simulink model "Model_TranslationEngine64"  (R2022b)
settings: Solver=FixedStepDiscrete  StartTime=0.0  StopTime=5  RelTol=1e-3  EnableMultiTasking=on
InitFcn:
  | % Initialize model
  | ModelSettings=BTConfig.GetModelSettings();
  | 
  | ModelSettings.Validate();
  | 
  | ModelInit;
  | 
  | 
  | % load library data
  | GainLibrary_data;
  | % Load saved values from partition process
  | CapturedConstMask.LoadMapFromFile(bdroot)
StartFcn:
  | % make sure all the simulated RTC requests are found
  | %RTC_SIM_OBJ.ValidateREQs();
undefined symbols (not defined in the file or in its folder): AA, BPLP, Column, NumHFRefBPF, NumHFRefLPF, NumMusicChannels, Row, VolumeMuteConfig
libraries: TuneVar x925, TOP x490, FeaturePath x111, CapturedConstLib x52
(part 18 of 34)

== system Model_TranslationEngine64/ModelPreAmp/DecRate/AudioPilot35/EntertainmentLevelDetection/AudiopilotLevelDetect/AudiopilotLevelDetect/HoldTime ==
  TOP : TOP/TOP  TriggerInit=[495 17 755 83]  TopName=HoldTimeSamples  DataTypeOut=single  BankNumber=0  PreOverlay=false  PostOverlay=false  Role=Automatic
      settings: SourceProductName=Bose Talaria
  TranslateTrigger : TuneVar/TranslateTrigger  TriggerInit=[306 -100 344 -45]
      settings: SourceProductName=Bose Talaria
  Tune Variable : TuneVar/TuneVar  TuneName=HoldTimeS  SpecifyMaxSize=off  VariableDim=1 (Row)  MaxSize=[1 1]  TunabilityNumber=1  MinValue=[]  MaxValue=[]  TriggerInit=[-115 17 145 83]  MaskValue=Config.HoldTimeSec
      settings: SourceProductName=Bose Talaria
  sec2samples : MATLAB Function  TreatAsAtomicUnit=on
  wires:
  TranslateTrigger/1 -> sec2samples/Trigger
  sec2samples/1(y) -> TOP/1
  Tune Variable/1 -> sec2samples/1(u)  "HoldTimeS"

== system Model_TranslationEngine64/ModelPreAmp/DecRate/AudioPilot35/EntertainmentLevelDetection/AudiopilotLevelDetect/AudiopilotLevelDetect/MaxVolume ==
  TOP : TOP/TOP  TriggerInit=[440 20 585 80]  TopName=MaxVolumeDb  DataTypeOut=single  BankNumber=BankNumber  PreOverlay=PreOverlay  PostOverlay=PostOverlay  Role=Automatic
      settings: SourceProductName=Bose Talaria
  TrivialTranslation : TuneVar/TrivialTranslation  TriggerInit=[300 28 350 72]
      settings: SourceProductName=Bose Talaria
  Tune Variable : TuneVar/TuneVar  TuneName=MaxVolumeDb  SpecifyMaxSize=off  VariableDim=1 (Row)  MaxSize=[1 1]  TunabilityNumber=1  MinValue=MinValue  MaxValue=MaxValue  TriggerInit=[20 25 190 75]  MaskValue=MaskValue
      settings: SourceProductName=Bose Talaria
  wires:
  Tune Variable/1 -> TrivialTranslation/1  "MaxVolumeDb"
  TrivialTranslation/1 -> TOP/1

== system Model_TranslationEngine64/ModelPreAmp/DecRate/AudioPilot35/EntertainmentLevelDetection/AudiopilotLevelDetect/AudiopilotLevelDetect/MinVolume ==
  TOP : TOP/TOP  TriggerInit=[440 20 585 80]  TopName=MinVolumeDb  DataTypeOut=single  BankNumber=BankNumber  PreOverlay=PreOverlay  PostOverlay=PostOverlay  Role=Automatic
      settings: SourceProductName=Bose Talaria
  TrivialTranslation : TuneVar/TrivialTranslation  TriggerInit=[300 28 350 72]
      settings: SourceProductName=Bose Talaria
  Tune Variable : TuneVar/TuneVar  TuneName=MinVolumeDb  SpecifyMaxSize=off  VariableDim=1 (Row)  MaxSize=[1 1]  TunabilityNumber=1  MinValue=MinValue  MaxValue=MaxValue  TriggerInit=[20 25 190 75]  MaskValue=MaskValue
      settings: SourceProductName=Bose Talaria
  wires:
  Tune Variable/1 -> TrivialTranslation/1  "MinVolumeDb"
  TrivialTranslation/1 -> TOP/1

== system Model_TranslationEngine64/ModelPreAmp/DecRate/AudioPilot35/EntertainmentLevelDetection/AudiopilotLevelDetect/AudiopilotLevelDetect/SlowDecay ==
  TOP : TOP/TOP  TriggerInit=[445 15 710 85]  TopName=SlowDecayDbPerSample  DataTypeOut=single  BankNumber=0  PreOverlay=false  PostOverlay=false  Role=Automatic
      settings: SourceProductName=Bose Talaria
  TranslateTrigger : TuneVar/TranslateTrigger  TriggerInit=[306 -100 344 -45]
      settings: SourceProductName=Bose Talaria
  Tune Variable : TuneVar/TuneVar  TuneName=SlowDecayDbPerS  SpecifyMaxSize=off  VariableDim=1 (Row)  MaxSize=[1 1]  TunabilityNumber=1  MinValue=[]  MaxValue=[]  TriggerInit=[-130 15 135 85]  MaskValue=Config.SlowDecayDbpersec
      settings: SourceProductName=Bose Talaria
  sec2samples : MATLAB Function  TreatAsAtomicUnit=on
  wires:
  TranslateTrigger/1 -> sec2samples/Trigger
  sec2samples/1(y) -> TOP/1
  Tune Variable/1 -> sec2samples/1(u)  "SlowDecayDbPerS"

== system Model_TranslationEngine64/ModelPreAmp/DecRate/AudioPilot35/EntertainmentLevelDetection/DyneqLevelDetect/DyneqLevelDetect/FastDecay ==
  TOP : TOP/TOP  TriggerInit=[495 17 745 83]  TopName=FastDecayDbPerSample  DataTypeOut=single  BankNumber=0  PreOverlay=false  PostOverlay=false  Role=Automatic
      settings: SourceProductName=Bose Talaria
  TranslateTrigger : TuneVar/TranslateTrigger  TriggerInit=[306 -100 344 -45]
      settings: SourceProductName=Bose Talaria
  Tune Variable : TuneVar/TuneVar  TuneName=FastDecayDbPerS  SpecifyMaxSize=off  VariableDim=1 (Row)  MaxSize=[1 1]  TunabilityNumber=1  MinValue=[]  MaxValue=[]  TriggerInit=[-155 17 95 83]  MaskValue=Config.FastDecayDbpersec
      settings: SourceProductName=Bose Talaria
  sec2samples : MATLAB Function  TreatAsAtomicUnit=on
  wires:
  TranslateTrigger/1 -> sec2samples/Trigger
  sec2samples/1(y) -> TOP/1
  Tune Variable/1 -> sec2samples/1(u)  "FastDecayDbPerS"

== system Model_TranslationEngine64/ModelPreAmp/DecRate/AudioPilot35/EntertainmentLevelDetection/DyneqLevelDetect/DyneqLevelDetect/HoldMargin ==
  SetPositive : MATLAB Function  TreatAsAtomicUnit=on
  TOP : TOP/TOP  TriggerInit=[440 20 640 80]  TopName=HoldMarginDb  DataTypeOut=single  BankNumber=0  PreOverlay=false  PostOverlay=false  Role=Automatic
      settings: SourceProductName=Bose Talaria
  TranslateTrigger : TuneVar/TranslateTrigger  TriggerInit=[306 -100 344 -45]
      settings: SourceProductName=Bose Talaria
  Tune Variable : TuneVar/TuneVar  TuneName=HoldMarginDb  SpecifyMaxSize=off  VariableDim=1 (Row)  MaxSize=[1 1]  TunabilityNumber=1  MinValue=[]  MaxValue=[]  TriggerInit=[-120 22 90 78]  MaskValue=Config.HoldMarginDb
      settings: SourceProductName=Bose Talaria
  wires:
  Tune Variable/1 -> SetPositive/1(Tune)  "HoldMarginDb"
  SetPositive/1(TOP) -> TOP/1
  TranslateTrigger/1 -> SetPositive/Trigger

== system Model_TranslationEngine64/ModelPreAmp/DecRate/AudioPilot35/EntertainmentLevelDetection/DyneqLevelDetect/DyneqLevelDetect/HoldTime ==
  TOP : TOP/TOP  TriggerInit=[475 15 725 85]  TopName=HoldTimeSamples  DataTypeOut=single  BankNumber=0  PreOverlay=false  PostOverlay=false  Role=Automatic
      settings: SourceProductName=Bose Talaria
  TranslateTrigger : TuneVar/TranslateTrigger  TriggerInit=[306 -100 344 -45]
      settings: SourceProductName=Bose Talaria
  Tune Variable : TuneVar/TuneVar  TuneName=HoldTimeS  SpecifyMaxSize=off  VariableDim=1 (Row)  MaxSize=[1 1]  TunabilityNumber=1  MinValue=[]  MaxValue=[]  TriggerInit=[-110 15 140 85]  MaskValue=Config.HoldTimeSec
      settings: SourceProductName=Bose Talaria
  sec2samples : MATLAB Function  TreatAsAtomicUnit=on
  wires:
  TranslateTrigger/1 -> sec2samples/Trigger
  sec2samples/1(y) -> TOP/1
  Tune Variable/1 -> sec2samples/1(u)  "HoldTimeS"

== system Model_TranslationEngine64/ModelPreAmp/DecRate/AudioPilot35/EntertainmentLevelDetection/DyneqLevelDetect/DyneqLevelDetect/MaxVolume ==
  TOP : TOP/TOP  TriggerInit=[440 20 585 80]  TopName=MaxVolumeDb  DataTypeOut=single  BankNumber=BankNumber  PreOverlay=PreOverlay  PostOverlay=PostOverlay  Role=Automatic
      settings: SourceProductName=Bose Talaria
  TrivialTranslation : TuneVar/TrivialTranslation  TriggerInit=[300 28 350 72]
      settings: SourceProductName=Bose Talaria
  Tune Variable : TuneVar/TuneVar  TuneName=MaxVolumeDb  SpecifyMaxSize=off  VariableDim=1 (Row)  MaxSize=[1 1]  TunabilityNumber=1  MinValue=MinValue  MaxValue=MaxValue  TriggerInit=[20 25 190 75]  MaskValue=MaskValue
      settings: SourceProductName=Bose Talaria
  wires:
  Tune Variable/1 -> TrivialTranslation/1  "MaxVolumeDb"
  TrivialTranslation/1 -> TOP/1

== system Model_TranslationEngine64/ModelPreAmp/DecRate/AudioPilot35/EntertainmentLevelDetection/DyneqLevelDetect/DyneqLevelDetect/MinVolume ==
  TOP : TOP/TOP  TriggerInit=[440 20 585 80]  TopName=MinVolumeDb  DataTypeOut=single  BankNumber=BankNumber  PreOverlay=PreOverlay  PostOverlay=PostOverlay  Role=Automatic
      settings: SourceProductName=Bose Talaria
  TrivialTranslation : TuneVar/TrivialTranslation  TriggerInit=[300 28 350 72]
      settings: SourceProductName=Bose Talaria
  Tune Variable : TuneVar/TuneVar  TuneName=MinVolumeDb  SpecifyMaxSize=off  VariableDim=1 (Row)  MaxSize=[1 1]  TunabilityNumber=1  MinValue=MinValue  MaxValue=MaxValue  TriggerInit=[20 25 190 75]  MaskValue=MaskValue
      settings: SourceProductName=Bose Talaria
  wires:
  Tune Variable/1 -> TrivialTranslation/1  "MinVolumeDb"
  TrivialTranslation/1 -> TOP/1

== system Model_TranslationEngine64/ModelPreAmp/DecRate/AudioPilot35/EntertainmentLevelDetection/DyneqLevelDetect/DyneqLevelDetect/SlowDecay ==
  TOP : TOP/TOP  TriggerInit=[440 17 695 83]  TopName=SlowDecayDbPerSample  DataTypeOut=single  BankNumber=0  PreOverlay=false  PostOverlay=false  Role=Automatic
      settings: SourceProductName=Bose Talaria
  TranslateTrigger : TuneVar/TranslateTrigger  TriggerInit=[306 -100 344 -45]
      settings: SourceProductName=Bose Talaria
  Tune Variable : TuneVar/TuneVar  TuneName=SlowDecayDbPerS  SpecifyMaxSize=off  VariableDim=1 (Row)  MaxSize=[1 1]  TunabilityNumber=1  MinValue=[]  MaxValue=[]  TriggerInit=[-115 17 140 83]  MaskValue=Config.SlowDecayDbpersec
      settings: SourceProductName=Bose Talaria
  sec2samples : MATLAB Function  TreatAsAtomicUnit=on
  wires:
  TranslateTrigger/1 -> sec2samples/Trigger
  sec2samples/1(y) -> TOP/1
  Tune Variable/1 -> sec2samples/1(u)  "SlowDecayDbPerS"

== system Model_TranslationEngine64/ModelPreAmp/DecRate/AudioPilot35/EntertainmentLevelDetection/PreProcessing/PreEmphasisShelfFilter/InnerLink ==
  PoolIirTunableWithReset : Subsystem  mask(Bose Pool IIR Tunable){FeatureName=Preemphasis, Config=Config}
      mask prompts: FeatureName "Filter name/purpose"; Config "PoolIirTunableWithResetConfig"
      mask help:
      | Pool IIR Tunable is a configurable multi-channel IIR filter that supports one or more channels. This block offers flexibility of tuning the number of stages and coefficients. Different filter coefficients and number of stages (biquads) can be used for each channel filter. The Pool IIR Tunable block supports different implementations, which could be configured at build-time:
      |
      | (i)   Generic: IIR filter code not optimized for any processor
      | (ii)  SharcCore: IIR filters executing on core (uses pooliir.asm CRL)
      | (iii) SharcGulAccel: IIR filters executing on IIR hardware accelerator, offloading MIPS usage from core
      | (iv) SharcGxpAccel: IIR filters take advantage of additional accelerators available on GXP processor
      | (v)  Hexagon: TBD
      |
      | NOTE: When using Pool IIR for Sharc-plus based processors, the codeWorkMemory buffer and input buffer should always be mapped to L1 memory to optimize MIPS utilization and avoid audio artifacts.
      |
      | For more information, please see 'Help'.
      mask init:
      | blkh=gcbh;
      | Config=BTConfig.Assert(blkh,Config);
      | 
      | BTConfig.InitSetFeatureIfPresent(blkh,'FeatureName');
      | Config.Validate();
      | Config.DoMaskInit(blkh);
      mask Help:
      | <b>Input signals: </b>
      | AudioIn: input channels [frame size x number of channels]
      | ResetTrigger: trigger to reset internal state buffer (usually preferred as a post RMDL step)
      | 
      | <b>Output signals: </b>
      | AudioOut: output channels [frame size x number of channels]
      | 
      | <b>Mask parameters: </b>
      | PoolIirTunableWithResetConfig
      | Filter name/purpose
      mask TypeOptions FeatureName: FeaturePath/FeatureName
      mask Callback Config: BTConfig.CallbackHideIfPresent(gcbh,{'FeatureName'});
      mask Display: DrawPoolIirIcon;

== system Model_TranslationEngine64/ModelPreAmp/DecRate/Medusa5H1/MedusaHoligram/Medusa5H1 Part 1/Bass Manager Stereo/Bass Manager Tuning ==
  surroundOn : Inport
  LeftMixIns : TuneVar/TuneVar  TuneName=LeftMixWeights  SpecifyMaxSize=off  VariableDim=1 (Row)  MaxSize=[1 1]  TunabilityNumber=1  MinValue=0  MaxValue=[]  TriggerInit=[20 429 205 471]  MaskValue=Config.TuneDefaults.LeftMixWeights
      settings: SourceProductName=Bose Talaria
  LeftMixWeight : TOP/TOP  TriggerInit=[545 367 735 423]  TopName=LeftMixWeights  DataTypeOut=Inherit: Same as input  BankNumber=0  PreOverlay=false  PostOverlay=false  Role=Automatic
      settings: SourceProductName=Bose Talaria
  RightMixIns : TuneVar/TuneVar  TuneName=RightMixWeights  SpecifyMaxSize=off  VariableDim=1 (Row)  MaxSize=[1 1]  TunabilityNumber=1  MinValue=0  MaxValue=[]  TriggerInit=[20 504 205 546]  MaskValue=Config.TuneDefaults.RightMixWeights
      settings: SourceProductName=Bose Talaria
  RightMixWeight : TOP/TOP  TriggerInit=[545 477 735 533]  TopName=RightMixWeights  DataTypeOut=single  BankNumber=0  PreOverlay=false  PostOverlay=false  Role=Automatic
      settings: SourceProductName=Bose Talaria
  TranslateTrigger : TuneVar/TranslateTrigger  TriggerInit=[366 240 404 295]
      settings: SourceProductName=Bose Talaria
  translation : MATLAB Function  TreatAsAtomicUnit=on  mask{NumInputs=Config.NumInputs}
  wires:
  translation/2(RightMixWeights) -> RightMixWeight/1
  RightMixIns/1 -> translation/3(RightMixWeightsIn)  "RightMixWeights"
  LeftMixIns/1 -> translation/2(LeftMixWeightsIn)  "LeftMixWeights"
  translation/1(LeftMixWeights) -> LeftMixWeight/1
  TranslateTrigger/1 -> translation/Trigger
  surroundOn/1 -> translation/1(SurroundOn)

== system Model_TranslationEngine64/ModelPreAmp/DecRate/Medusa5H1/MedusaHoligram/Medusa5H1 Part 1/Bass Manager Stereo/HPF ==
  PoolIirTunableWithReset : Subsystem  mask(Bose Pool IIR Tunable){FeatureName=Hpf, Config=Config}
      mask prompts: FeatureName "Filter name/purpose"; Config "PoolIirTunableWithResetConfig"
      mask help:
      | Pool IIR Tunable is a configurable multi-channel IIR filter that supports one or more channels. This block offers flexibility of tuning the number of stages and coefficients. Different filter coefficients and number of stages (biquads) can be used for each channel filter. The Pool IIR Tunable block supports different implementations, which could be configured at build-time:
      |
      | (i)   Generic: IIR filter code not optimized for any processor
      | (ii)  SharcCore: IIR filters executing on core (uses pooliir.asm CRL)
      | (iii) SharcGulAccel: IIR filters executing on IIR hardware accelerator, offloading MIPS usage from core
      | (iv) SharcGxpAccel: IIR filters take advantage of additional accelerators available on GXP processor
      | (v)  Hexagon: TBD
      |
      | NOTE: When using Pool IIR for Sharc-plus based processors, the codeWorkMemory buffer and input buffer should always be mapped to L1 memory to optimize MIPS utilization and avoid audio artifacts.
      |
      | For more information, please see 'Help'.
      mask init:
      | blkh=gcbh;
      | Config=BTConfig.Assert(blkh,Config);
      | 
      | BTConfig.InitSetFeatureIfPresent(blkh,'FeatureName');
      | Config.Validate();
      | Config.DoMaskInit(blkh);
      mask Help:
      | <b>Input signals: </b>
      | AudioIn: input channels [frame size x number of channels]
      | ResetTrigger: trigger to reset internal state buffer (usually preferred as a post RMDL step)
      | 
      | <b>Output signals: </b>
      | AudioOut: output channels [frame size x number of channels]
      | 
      | <b>Mask parameters: </b>
      | PoolIirTunableWithResetConfig
      | Filter name/purpose
      mask TypeOptions FeatureName: FeaturePath/FeatureName
      mask Callback Config: BTConfig.CallbackHideIfPresent(gcbh,{'FeatureName'});
      mask Display: DrawPoolIirIcon;

== system Model_TranslationEngine64/ModelPreAmp/DecRate/Medusa5H1/MedusaHoligram/Medusa5H1 Part 1/Bass Manager Stereo/LPF ==
  PoolIirTunableWithReset : Subsystem  mask(Bose Pool IIR Tunable){FeatureName=Lpf, Config=Config}
      mask prompts: FeatureName "Filter name/purpose"; Config "PoolIirTunableWithResetConfig"
      mask help:
      | Pool IIR Tunable is a configurable multi-channel IIR filter that supports one or more channels. This block offers flexibility of tuning the number of stages and coefficients. Different filter coefficients and number of stages (biquads) can be used for each channel filter. The Pool IIR Tunable block supports different implementations, which could be configured at build-time:
      |
      | (i)   Generic: IIR filter code not optimized for any processor
      | (ii)  SharcCore: IIR filters executing on core (uses pooliir.asm CRL)
      | (iii) SharcGulAccel: IIR filters executing on IIR hardware accelerator, offloading MIPS usage from core
      | (iv) SharcGxpAccel: IIR filters take advantage of additional accelerators available on GXP processor
      | (v)  Hexagon: TBD
      |
      | NOTE: When using Pool IIR for Sharc-plus based processors, the codeWorkMemory buffer and input buffer should always be mapped to L1 memory to optimize MIPS utilization and avoid audio artifacts.
      |
      | For more information, please see 'Help'.
      mask init:
      | blkh=gcbh;
      | Config=BTConfig.Assert(blkh,Config);
      | 
      | BTConfig.InitSetFeatureIfPresent(blkh,'FeatureName');
      | Config.Validate();
      | Config.DoMaskInit(blkh);
      mask Help:
      | <b>Input signals: </b>
      | AudioIn: input channels [frame size x number of channels]
      | ResetTrigger: trigger to reset internal state buffer (usually preferred as a post RMDL step)
      | 
      | <b>Output signals: </b>
      | AudioOut: output channels [frame size x number of channels]
      | 
      | <b>Mask parameters: </b>
      | PoolIirTunableWithResetConfig
      | Filter name/purpose
      mask TypeOptions FeatureName: FeaturePath/FeatureName
      mask Callback Config: BTConfig.CallbackHideIfPresent(gcbh,{'FeatureName'});
      mask Display: DrawPoolIirIcon;

== system Model_TranslationEngine64/ModelPreAmp/DecRate/Medusa5H1/MedusaHoligram/Medusa5H1 Part 1/Bass Manager Stereo/TuneTOP ==
  TOP : TOP/TOP  TriggerInit=[440 20 585 80]  TopName=GainLfe2C  DataTypeOut=single  BankNumber=BankNumber  PreOverlay=PreOverlay  PostOverlay=PostOverlay  Role=Automatic
      settings: SourceProductName=Bose Talaria
  TrivialTranslation : TuneVar/TrivialTranslation  TriggerInit=[300 28 350 72]
      settings: SourceProductName=Bose Talaria
  Tune Variable : TuneVar/TuneVar  TuneName=GainLfe2C  SpecifyMaxSize=off  VariableDim=1 (Row)  MaxSize=[1 1]  TunabilityNumber=1  MinValue=MinValue  MaxValue=MaxValue  TriggerInit=[20 25 190 75]  MaskValue=MaskValue
      settings: SourceProductName=Bose Talaria
  wires:
  Tune Variable/1 -> TrivialTranslation/1  "GainLfe2C"
  TrivialTranslation/1 -> TOP/1

== system Model_TranslationEngine64/ModelPreAmp/DecRate/Medusa5H1/MedusaHoligram/Medusa5H1 Part 1/CAE Treble Boost/Audio Passthrough ==
  TuneTOP : Subsystem  mask(Talaria Trivial Tune TOP){TriggerInit=[50 262 220 318], TopName=DummyTune, TuneName=DummyTune, DataTypeOut=single, MaskValue=[1], TunabilityNumber=1, MinValue=[], MaxValue=[], BankNumber=0, PreOverlay=false, PostOverlay=false, UseSameName=on}
      mask prompts: TriggerInit "Hidden: MoveFcn redraw"; TopName "Name:"; TuneName "Name of TuneVar:"; DataTypeOut "Data type:"; MaskValue "Default Value:"; TunabilityNumber "Tunability:"; MinValue "Min Value:"; MaxValue "Max Value:"; BankNumber "Target memory bank number:"; PreOverlay "Requires pre-overlay action:"; PostOverlay "Requires post-overlay action:"; UseSameName "Use same name for tune variable and TOP"
      mask help: The TuneTOP block encapsultes a Target Overlay Parameter, a Tune Variable, and a Trivial Translation between them.
      mask init:
      | [ok,activeTopPath,activeTunePath] = TuneTOP_Mask.Init(gcbh);
      settings: MoveFcn=TuneTOP_Mask.CB_TriggerInit(gcbh);
      mask Callback TriggerInit: TuneTOP_Mask.CB_TriggerInit(gcbh);
      mask TypeOptions TopName: TOP/TopName
      mask TypeOptions TuneName: Tune Variable/TuneName
      mask TypeOptions DataTypeOut: TOP/DataTypeOut
      mask TypeOptions MaskValue: Tune Variable/MaskValue
      mask TypeOptions TunabilityNumber: Tune Variable/TunabilityNumber
      mask Callback TunabilityNumber: TuneVarMask.CB_TunabilityNumber(gcbh);
      mask TypeOptions MinValue: Tune Variable/MinValue
      mask TypeOptions MaxValue: Tune Variable/MaxValue
      mask TypeOptions BankNumber: TOP/BankNumber
      mask TypeOptions PreOverlay: TOP/PreOverlay
      mask TypeOptions PostOverlay: TOP/PostOverlay
      mask Callback UseSameName: TuneTOP_Mask.CB_UseSameName(gcbh);
      mask DialogControl toolPanel Prompt: Tuning Tool Hints
      mask DialogControl DescriptionGroup Prompt: Description
      mask DialogControl EditDescription Prompt: Edit Description
      mask DialogControl EditDescription Callback: TuneTOP_Mask.CB_EditDescription(gcbh);
      mask DialogControl TunabilityText Prompt: Easy: Changes nearly every tuning.
      mask DialogControl AdvancedPanel Prompt: Advanced
      mask DialogControl ConvertToFullTranslation Prompt: Irreversible conversion to full translation
      mask DialogControl ConvertToFullTranslation Callback: TuneTOP_Mask.CB_ConvertToFullTranslation(gcbh);
      mask DialogControl ErrorContainer Prompt: Error Messages
      mask Display:
      | % retrieve icon definition
      | [path,w,h] = TuneTOP_Mask.Icon();
      | 
      | % retrieve the block's pixel size
      | pos = get(gcbh,'position');
      | bw = pos(3) - pos(1);
      | bh = pos(4) - pos(2);
      | 
      | % draw centered icon
      | xAdj = bw/2 - w/2 + 5;
      | yAdj = bh/2 - h/2 + 4;
      | for i=1:length(path)
      | 	patch(path(i).x+xAdj, path(i).y+yAdj, path(i).rgb);
      | end
      | 
      | % show the top name or an X
      | if (exist('ok','var') && ok)
      | 	text(bw*0.5, bh*0.2, activeTopPath, 'horizontalAlignment', 'center');
      | 	patch(0,0,[1 1 1]);
      | 	patch(bw,bh,[1 1 1]);
      | else
      | 	tx=bw*0.03;
      | 	ty=bh*0.03;
      | 	patch([0 tx bw bw-tx], [ty 0 bh-ty bh], [1 0 0]);
      | 	patch([0 bw-tx bw tx], [bh-ty 0 ty bh], [1 0 0]);
      | end

== system Model_TranslationEngine64/ModelPreAmp/DecRate/Medusa5H1/MedusaHoligram/Medusa5H1 Part 1/CAE Treble Boost/CAE Treble Boost ==

== system Model_TranslationEngine64/ModelPreAmp/DecRate/Medusa5H1/MedusaHoligram/Medusa5H1 Part 2/Alignment Delay/Full-rate Alignment Delay Translation ==
  DeciRateWiggleDelaySamples : Inport
  DeciRateNearWiggleDelaySamples : Inport  Port=2
  HoligramDelaySamples : Inport  Port=3
  TranslateTrigger : TuneVar/TranslateTrigger  TriggerInit=[211 55 249 110]
      settings: SourceProductName=Bose Talaria
  Treble Delay : TOP/TOP  TriggerInit=[355 205 500 265]  TopName=TrebleDelay  DataTypeOut=int32  BankNumber=0  PreOverlay=false  PostOverlay=false  Role=Automatic
      settings: SourceProductName=Bose Talaria
  translation : MATLAB Function  TreatAsAtomicUnit=on  mask{DecimationFactor=Config.DecimationFactor, DeciRateMaxWiggleDelay=Config.DeciRateMaxWiggleDelay, DeciRateMaxNearWiggleDelay=Config.DeciRateMaxNearWiggleDelay, MaxHoligramDelay=Config.MaxHoligramDelay, DeciRateFdpDelay=Config.DeciRateFdpDelay, FullRateFdpDelay=Config.FullRateFdpDelay, MaxTrebleDelay=Config.MaxTrebleDelay}
  wires:
  DeciRateNearWiggleDelaySamples/1 -> translation/2(NEARWiggleDelay)
  DeciRateWiggleDelaySamples/1 -> translation/1(wiggleDelay)
  TranslateTrigger/1 -> translation/Trigger
  translation/1(trebleDelay) -> Treble Delay/1
  HoligramDelaySamples/1 -> translation/3(holigramDelay)

== system Model_TranslationEngine64/ModelPreAmp/DecRate/Medusa5H1/MedusaHoligram/Medusa5H1 Part 2/Decimated-Rate FDP/Fdp ==
  FeaturePath : FeaturePath/FeaturePath  FeatureName=Fdp  IsGroup=off  GroupNumber=-1  IsModule=off  TriggerInit=[260 -121 375 -14]
      settings: SourceProductName=Bose Talaria
  FreqDomainProcessing : Subsystem
  Goto Tag Visibility : GotoTagVisibility  GotoTag=LsSmooth
  Goto Tag Visibility1 : GotoTagVisibility  GotoTag=DirectPathSec
  Goto Tag Visibility2 : GotoTagVisibility  GotoTag=FastPsdSmoothCutoff
  Goto Tag Visibility3 : GotoTagVisibility  GotoTag=SlowPsdSmoothCutoff
  Goto Tag Visibility6 : GotoTagVisibility  GotoTag=deciRateXpMax
  Tune Variable : TuneVar/TuneVar  Description=Cutoff frequeny for single pole averager that smooths slow PSD used in SPUM.  TuneName=SlowPsdSmoothCutoff  SpecifyMaxSize=off  VariableDim=1 (Row)  MaxSize=[1 1]  TunabilityNumber=2  MinValue=[]  MaxValue=[]  TriggerInit=[240 485 410 535]  MaskValue=Config.TuneDefaults.FdpSlowPsdSmoothCutoff
      settings: SourceProductName=Bose Talaria
  Tune Variable1 : TuneVar/TuneVar  Description=Cutoff frequeny for single pole averager that smooths fast PSD used in SPUM.  TuneName=FastPsdSmoothCutoff  SpecifyMaxSize=off  VariableDim=1 (Row)  MaxSize=[1 1]  TunabilityNumber=2  MinValue=[]  MaxValue=[]  TriggerInit=[240 550 410 600]  MaskValue=Config.TuneDefaults.FdpFastPsdSmoothCutoff
      settings: SourceProductName=Bose Talaria
  Tune Variable2 : TuneVar/TuneVar  Description=This is the time in seconds that separates dry (or direct) and reverb parts. The larger directPathSec becomes, the more energy goes into the “impulse” because a longer period of time past “onset” is considered direct energy. Ideally this value is equivalent to an integer multiple of a frame period.  TuneName=DirectPathSec  SpecifyMaxSize=off  VariableDim=1 (Row)  MaxSize=[1 1]  TunabilityNumber=2  MinValue=[]  MaxValue=[]  TriggerInit=[240 680 410 730]  MaskValue=Config.TuneDefaults.FdpDirectPathSec
      settings: SourceProductName=Bose Talaria
  Tune Variable3 : TuneVar/TuneVar  Description=Cutoff frequency for lowpass filter that is used to smooth Hreverb and energy used in SPUM.  TuneName=LsSmoothCutoff  SpecifyMaxSize=off  VariableDim=1 (Row)  MaxSize=[1 1]  TunabilityNumber=2  MinValue=[]  MaxValue=[]  TriggerInit=[240 615 410 665]  MaskValue=Config.TuneDefaults.FdpLsSmoothCutoff
      settings: SourceProductName=Bose Talaria
  Tune Variable7 : TuneVar/TuneVar  Description=Minimum stretch factor - must be in range [0,1)  TuneName=XpMax  SpecifyMaxSize=off  VariableDim=1 (Row)  MaxSize=[1 1]  TunabilityNumber=1  MinValue=0  MaxValue=1  TriggerInit=[240 420 405 470]  MaskValue=Config.TuneDefaults.FdpDeciRateXpMax
      settings: SourceProductName=Bose Talaria
  TuneTOP : Subsystem  Description=|  mask(Talaria Trivial Tune TOP){TriggerInit=[240 747 410 803], TopName=SpumOverwrite, TuneName=SpumOverwrite, DataTypeOut=single, MaskValue=Config.TuneDefaults.FdpSpumOverwrite, TunabilityNumber=3, MinValue=[], MaxValue=[], BankNumber=0, PreOverlay=false, PostOverlay=false, UseSameName=on}
      | This parameter overwrites the decay rate if needed for testing purposes. The valid options are:
      | 0 (default): no overwrite
      | 1: all mono contents go to tail signals
      mask prompts: TriggerInit "Hidden: MoveFcn redraw"; TopName "Name:"; TuneName "Name of TuneVar:"; DataTypeOut "Data type:"; MaskValue "Default Value:"; TunabilityNumber "Tunability:"; MinValue "Min Value:"; MaxValue "Max Value:"; BankNumber "Target memory bank number:"; PreOverlay "Requires pre-overlay action:"; PostOverlay "Requires post-overlay action:"; UseSameName "Use same name for tune variable and TOP"
      mask help: The TuneTOP block encapsultes a Target Overlay Parameter, a Tune Variable, and a Trivial Translation between them.
      mask init:
      | [ok,activeTopPath,activeTunePath] = TuneTOP_Mask.Init(gcbh);
      settings: MoveFcn=TuneTOP_Mask.CB_TriggerInit(gcbh);
      mask Callback TriggerInit: TuneTOP_Mask.CB_TriggerInit(gcbh);
      mask TypeOptions TopName: TOP/TopName
      mask TypeOptions TuneName: Tune Variable/TuneName
      mask TypeOptions DataTypeOut: TOP/DataTypeOut
      mask TypeOptions MaskValue: Tune Variable/MaskValue
      mask TypeOptions TunabilityNumber: Tune Variable/TunabilityNumber
      mask Callback TunabilityNumber: TuneVarMask.CB_TunabilityNumber(gcbh);
      mask TypeOptions MinValue: Tune Variable/MinValue
      mask TypeOptions MaxValue: Tune Variable/MaxValue
      mask TypeOptions BankNumber: TOP/BankNumber
      mask TypeOptions PreOverlay: TOP/PreOverlay
      mask TypeOptions PostOverlay: TOP/PostOverlay
      mask Callback UseSameName: TuneTOP_Mask.CB_UseSameName(gcbh);
      mask DialogControl toolPanel Prompt: Tuning Tool Hints
      mask DialogControl DescriptionGroup Prompt: Description
      mask DialogControl EditDescription Prompt: Edit Description
      mask DialogControl EditDescription Callback: TuneTOP_Mask.CB_EditDescription(gcbh);
      mask DialogControl TunabilityText Prompt: Easy: Changes nearly every tuning.
      mask DialogControl AdvancedPanel Prompt: Advanced
      mask DialogControl ConvertToFullTranslation Prompt: Irreversible conversion to full translation
      mask DialogControl ConvertToFullTranslation Callback: TuneTOP_Mask.CB_ConvertToFullTranslation(gcbh);
      mask DialogControl ErrorContainer Prompt: Error Messages
      mask Display:
      | % retrieve icon definition
      | [path,w,h] = TuneTOP_Mask.Icon();
      | 
      | % retrieve the block's pixel size
      | pos = get(gcbh,'position');
      | bw = pos(3) - pos(1);
      | bh = pos(4) - pos(2);
      | 
      | % draw centered icon
      | xAdj = bw/2 - w/2 + 5;
      | yAdj = bh/2 - h/2 + 4;
      | for i=1:length(path)
      | 	patch(path(i).x+xAdj, path(i).y+yAdj, path(i).rgb);
      | end
      | 
      | % show the top name or an X
      | if (exist('ok','var') && ok)
      | 	text(bw*0.5, bh*0.2, activeTopPath, 'horizontalAlignment', 'center');
      | 	patch(0,0,[1 1 1]);
      | 	patch(bw,bh,[1 1 1]);
      | else
      | 	tx=bw*0.03;
      | 	ty=bh*0.03;
      | 	patch([0 tx bw bw-tx], [ty 0 bh-ty bh], [1 0 0]);
      | 	patch([0 bw-tx bw tx], [bh-ty 0 ty bh], [1 0 0]);
      | end
  tag scope: DirectPathSec=scoped, FastPsdSmoothCutoff=scoped, LsSmooth=scoped, SlowPsdSmoothCutoff=scoped, deciRateXpMax=scoped
  wires:
  Tune Variable7/1 -> [deciRateXpMax]  "XpMax"
  Tune Variable/1 -> [SlowPsdSmoothCutoff]  "SlowPsdSmoothCutoff"
  Tune Variable1/1 -> [FastPsdSmoothCutoff]  "FastPsdSmoothCutoff"
  Tune Variable3/1 -> [LsSmooth]  "LsSmoothCutoff"
  Tune Variable2/1 -> [DirectPathSec]  "DirectPathSec"

== system Model_TranslationEngine64/ModelPreAmp/DecRate/Medusa5H1/MedusaHoligram/Medusa5H1 Part 2/Full-Rate FDP/Fdp ==
  FeaturePath : FeaturePath/FeaturePath  FeatureName=Fdp  IsGroup=off  GroupNumber=-1  IsModule=off  TriggerInit=[260 -121 375 -14]
      settings: SourceProductName=Bose Talaria
  FreqDomainProcessing : Subsystem
  Goto Tag Visibility : GotoTagVisibility  GotoTag=LsSmooth
  Goto Tag Visibility1 : GotoTagVisibility  GotoTag=DirectPathSec
  Goto Tag Visibility2 : GotoTagVisibility  GotoTag=FastPsdSmoothCutoff
  Goto Tag Visibility3 : GotoTagVisibility  GotoTag=SlowPsdSmoothCutoff
  Goto Tag Visibility6 : GotoTagVisibility  GotoTag=deciRateXpMax
  Tune Variable : TuneVar/TuneVar  Description=Cutoff frequeny for single pole averager that smooths slow PSD used in SPUM.  TuneName=SlowPsdSmoothCutoff  SpecifyMaxSize=off  VariableDim=1 (Row)  MaxSize=[1 1]  TunabilityNumber=2  MinValue=[]  MaxValue=[]  TriggerInit=[240 485 410 535]  MaskValue=Config.TuneDefaults.FdpSlowPsdSmoothCutoff
      settings: SourceProductName=Bose Talaria
  Tune Variable1 : TuneVar/TuneVar  Description=Cutoff frequeny for single pole averager that smooths fast PSD used in SPUM.  TuneName=FastPsdSmoothCutoff  SpecifyMaxSize=off  VariableDim=1 (Row)  MaxSize=[1 1]  TunabilityNumber=2  MinValue=[]  MaxValue=[]  TriggerInit=[240 550 410 600]  MaskValue=Config.TuneDefaults.FdpFastPsdSmoothCutoff
      settings: SourceProductName=Bose Talaria
  Tune Variable2 : TuneVar/TuneVar  Description=This is the time in seconds that separates dry (or direct) and reverb parts. The larger directPathSec becomes, the more energy goes into the “impulse” because a longer period of time past “onset” is considered direct energy. Ideally this value is equivalent to an integer multiple of a frame period.  TuneName=DirectPathSec  SpecifyMaxSize=off  VariableDim=1 (Row)  MaxSize=[1 1]  TunabilityNumber=2  MinValue=[]  MaxValue=[]  TriggerInit=[240 680 410 730]  MaskValue=Config.TuneDefaults.FdpDirectPathSec
      settings: SourceProductName=Bose Talaria
  Tune Variable3 : TuneVar/TuneVar  Description=Cutoff frequency for lowpass filter that is used to smooth Hreverb and energy used in SPUM.  TuneName=LsSmoothCutoff  SpecifyMaxSize=off  VariableDim=1 (Row)  MaxSize=[1 1]  TunabilityNumber=2  MinValue=[]  MaxValue=[]  TriggerInit=[240 615 410 665]  MaskValue=Config.TuneDefaults.FdpLsSmoothCutoff
      settings: SourceProductName=Bose Talaria
  Tune Variable7 : TuneVar/TuneVar  Description=Minimum stretch factor - must be in range [0,1)  TuneName=XpMax  SpecifyMaxSize=off  VariableDim=1 (Row)  MaxSize=[1 1]  TunabilityNumber=1  MinValue=0  MaxValue=1  TriggerInit=[240 420 405 470]  MaskValue=Config.TuneDefaults.FdpDeciRateXpMax
      settings: SourceProductName=Bose Talaria
  TuneTOP : Subsystem  Description=|  mask(Talaria Trivial Tune TOP){TriggerInit=[240 747 410 803], TopName=SpumOverwrite, TuneName=SpumOverwrite, DataTypeOut=single, MaskValue=Config.TuneDefaults.FdpSpumOverwrite, TunabilityNumber=3, MinValue=[], MaxValue=[], BankNumber=0, PreOverlay=false, PostOverlay=false, UseSameName=on}
      | This parameter overwrites the decay rate if needed for testing purposes. The valid options are:
      | 0 (default): no overwrite
      | 1: all mono contents go to tail signals
      mask prompts: TriggerInit "Hidden: MoveFcn redraw"; TopName "Name:"; TuneName "Name of TuneVar:"; DataTypeOut "Data type:"; MaskValue "Default Value:"; TunabilityNumber "Tunability:"; MinValue "Min Value:"; MaxValue "Max Value:"; BankNumber "Target memory bank number:"; PreOverlay "Requires pre-overlay action:"; PostOverlay "Requires post-overlay action:"; UseSameName "Use same name for tune variable and TOP"
      mask help: The TuneTOP block encapsultes a Target Overlay Parameter, a Tune Variable, and a Trivial Translation between them.
      mask init:
      | [ok,activeTopPath,activeTunePath] = TuneTOP_Mask.Init(gcbh);
      settings: MoveFcn=TuneTOP_Mask.CB_TriggerInit(gcbh);
      mask Callback TriggerInit: TuneTOP_Mask.CB_TriggerInit(gcbh);
      mask TypeOptions TopName: TOP/TopName
      mask TypeOptions TuneName: Tune Variable/TuneName
      mask TypeOptions DataTypeOut: TOP/DataTypeOut
      mask TypeOptions MaskValue: Tune Variable/MaskValue
      mask TypeOptions TunabilityNumber: Tune Variable/TunabilityNumber
      mask Callback TunabilityNumber: TuneVarMask.CB_TunabilityNumber(gcbh);
      mask TypeOptions MinValue: Tune Variable/MinValue
      mask TypeOptions MaxValue: Tune Variable/MaxValue
      mask TypeOptions BankNumber: TOP/BankNumber
      mask TypeOptions PreOverlay: TOP/PreOverlay
      mask TypeOptions PostOverlay: TOP/PostOverlay
      mask Callback UseSameName: TuneTOP_Mask.CB_UseSameName(gcbh);
      mask DialogControl toolPanel Prompt: Tuning Tool Hints
      mask DialogControl DescriptionGroup Prompt: Description
      mask DialogControl EditDescription Prompt: Edit Description
      mask DialogControl EditDescription Callback: TuneTOP_Mask.CB_EditDescription(gcbh);
      mask DialogControl TunabilityText Prompt: Easy: Changes nearly every tuning.
      mask DialogControl AdvancedPanel Prompt: Advanced
      mask DialogControl ConvertToFullTranslation Prompt: Irreversible conversion to full translation
      mask DialogControl ConvertToFullTranslation Callback: TuneTOP_Mask.CB_ConvertToFullTranslation(gcbh);
      mask DialogControl ErrorContainer Prompt: Error Messages
      mask Display:
      | % retrieve icon definition
      | [path,w,h] = TuneTOP_Mask.Icon();
      | 
      | % retrieve the block's pixel size
      | pos = get(gcbh,'position');
      | bw = pos(3) - pos(1);
      | bh = pos(4) - pos(2);
      | 
      | % draw centered icon
      | xAdj = bw/2 - w/2 + 5;
      | yAdj = bh/2 - h/2 + 4;
      | for i=1:length(path)
      | 	patch(path(i).x+xAdj, path(i).y+yAdj, path(i).rgb);
      | end
      | 
      | % show the top name or an X
      | if (exist('ok','var') && ok)
      | 	text(bw*0.5, bh*0.2, activeTopPath, 'horizontalAlignment', 'center');
      | 	patch(0,0,[1 1 1]);
      | 	patch(bw,bh,[1 1 1]);
      | else
      | 	tx=bw*0.03;
      | 	ty=bh*0.03;
      | 	patch([0 tx bw bw-tx], [ty 0 bh-ty bh], [1 0 0]);
      | 	patch([0 bw-tx bw tx], [bh-ty 0 ty bh], [1 0 0]);
      | end
  tag scope: DirectPathSec=scoped, FastPsdSmoothCutoff=scoped, LsSmooth=scoped, SlowPsdSmoothCutoff=scoped, deciRateXpMax=scoped
  wires:
  Tune Variable7/1 -> [deciRateXpMax]  "XpMax"
  Tune Variable/1 -> [SlowPsdSmoothCutoff]  "SlowPsdSmoothCutoff"
  Tune Variable1/1 -> [FastPsdSmoothCutoff]  "FastPsdSmoothCutoff"
  Tune Variable3/1 -> [LsSmooth]  "LsSmoothCutoff"
  Tune Variable2/1 -> [DirectPathSec]  "DirectPathSec"

== system Model_TranslationEngine64/ModelPreAmp/DecRate/Medusa5H1/MedusaHoligram/Medusa5H1 Part 2/Mono Detector/Mono Detector ==
  Tune Translations : Subsystem

== system Model_TranslationEngine64/ModelPreAmp/DecRate/Medusa5H1/MedusaHoligram/Medusa5H1 Part 2/Mono Detector/TuneTOP ==
  TOP : TOP/TOP  TriggerInit=[440 20 585 80]  TopName=Enable  DataTypeOut=int32  BankNumber=BankNumber  PreOverlay=PreOverlay  PostOverlay=PostOverlay  Role=Automatic
      settings: SourceProductName=Bose Talaria
  TrivialTranslation : TuneVar/TrivialTranslation  TriggerInit=[300 28 350 72]
      settings: SourceProductName=Bose Talaria
  Tune Variable : TuneVar/TuneVar  TuneName=Enable  SpecifyMaxSize=off  VariableDim=1 (Row)  MaxSize=[1 1]  TunabilityNumber=1  MinValue=MinValue  MaxValue=MaxValue  TriggerInit=[20 25 190 75]  MaskValue=MaskValue
      settings: SourceProductName=Bose Talaria
  wires:
  Tune Variable/1 -> TrivialTranslation/1  "Enable"
  TrivialTranslation/1 -> TOP/1
